simulink model "UKF_MPCwithDISTandRefer"  (R2016a)
settings: Solver=ode3  SolverMode=SingleTasking  StartTime=0.0  StopTime=32400  FixedStep=Ts  RelTol=1e-3
values from neighbouring files (symbols this model uses):
  R = log(D_ins_out / D_pipe) / (2 * pi * K * L/segments)    [Custom_pipe.m]    (also in ini_pipe_detailed.m = log(D_ins_out / D_pipe) / (2 * pi* K * L/segments))
undefined symbols (not defined in the file or in its folder): Nc, P_0, Q, Ts, x0_plant, x_s0, y_max, y_min
settings Model: Creator=saif  LastModifiedBy=lenovo
settings DataIOCC: LimitDataPoints=on  SaveFormat=Array
settings OptimizationCC: BlockReduction=off  BooleanDataType=off
settings DebuggingCC: SaveWithParameterizedLinksMsg=none  UnderspecifiedInitializationDetection=Classic  MergeDetectMultiDrivingBlocksExec=none  SignalResolutionControl=TryResolveAllWithWarning
settings HardwareCC: ProdBitPerPointer=32  ProdLargestAtomicFloat=None  ProdIntDivRoundTo=Undefined  ProdEndianess=Unspecified  ProdWordSize=32  ProdHWDeviceType=32-bit Generic  TargetUnknown=on
settings ModelReferenceCC: PropagateSignalLabelsOutOfModel=off
settings ConfigComp: CovModelRefEnable=Off  CovSFcnEnable=off

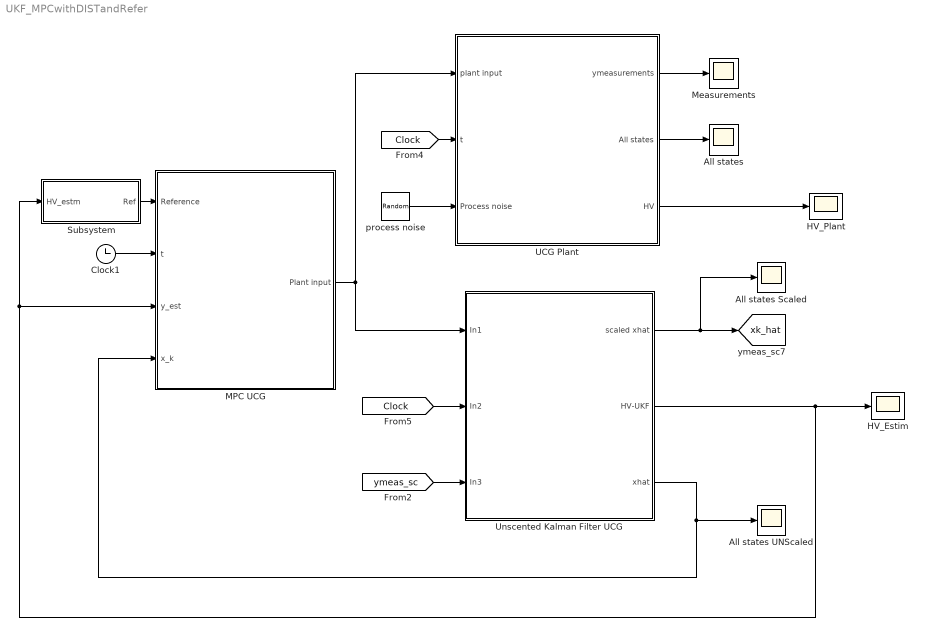
== system UKF_MPCwithDISTandRefer ==
  All states : Scope
  All states Scaled : Scope
  All states UNScaled : Scope
  Clock1 : Clock
  HV_Estim : Scope
  HV_Plant : Scope
  MPC UCG : Subsystem
  Measurements : Scope
  Subsystem : Subsystem
  UCG Plant : Subsystem
  Unscented Kalman Filter UCG : Subsystem
  process noise : RandomNumber  Variance=1e-4  SampleTime=Ts
  tag scope: xk_hat=global
  wires:
  process noise/1 -> UCG Plant/3(Process noise)
  UCG Plant/1(ymeasurements) -> Measurements/1
  UCG Plant/2(All states) -> All states/1
  Unscented Kalman Filter UCG/1(scaled xhat) -> All states Scaled/1, [xk_hat]
  Subsystem/1(Ref) -> MPC UCG/1(Reference)
  Clock1/1 -> MPC UCG/2(t)
  [Clock] -> UCG Plant/2(t)
  [Clock] -> Unscented Kalman Filter UCG/2(In2)
  UCG Plant/3(HV) -> HV_Plant/1
  Unscented Kalman Filter UCG/2(HV-UKF) -> Subsystem/1(HV_estm), MPC UCG/3(y_est), HV_Estim/1
  Unscented Kalman Filter UCG/3(xhat) -> All states UNScaled/1, MPC UCG/4(x_k)
  MPC UCG/1(Plant input) -> UCG Plant/1(plant input), Unscented Kalman Filter UCG/1(In1)
  [ymeas_sc] -> Unscented Kalman Filter UCG/3(In3)

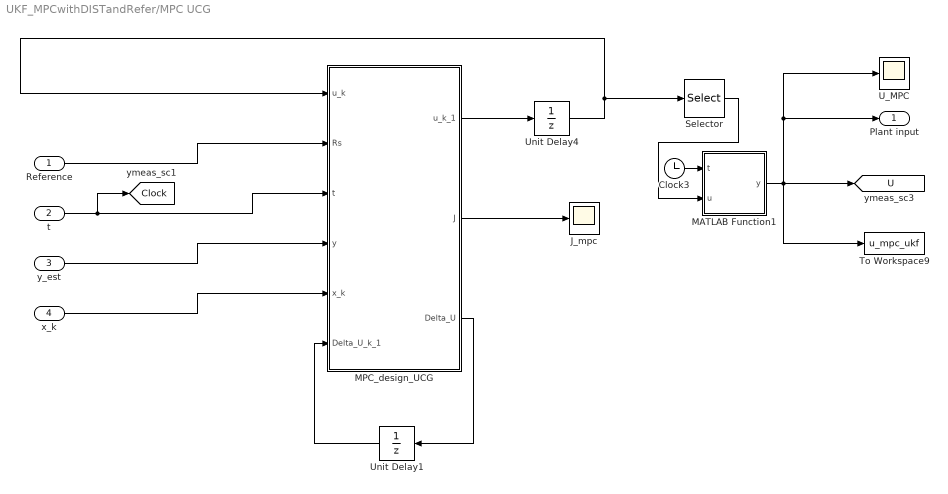
== system UKF_MPCwithDISTandRefer/MPC UCG ==
  Reference : Inport
  t : Inport  Port=2
  y_est : Inport  Port=3
  x_k : Inport  Port=4
  Clock3 : Clock
  J_mpc : Scope
  MATLAB Function1 : MATLAB Function  TreatAsAtomicUnit=on
  MPC_design_UCG : MATLAB Function  TreatAsAtomicUnit=on
  Selector : Selector  InputPortWidth=Nc  IndexOptions=Index vector (dialog)  Indices=[1]  OutputSizes=1
  To Workspace9 : ToWorkspace  VariableName=u_mpc_ukf  SampleTime=-1
  U_MPC : Scope
  Unit Delay1 : UnitDelay  InitialCondition=2e-4*ones(Nc,1)  SampleTime=-1
  Unit Delay4 : UnitDelay  InitialCondition=2e-4*ones(Nc,1)  SampleTime=-1
  Plant input : Outport
  tag scope: Clock=global, U=global
  wires:
  MATLAB Function1/1(y) -> To Workspace9/1, U_MPC/1, Plant input/1, [U]
  MPC_design_UCG/1(u_k_1) -> Unit Delay4/1
  Unit Delay4/1 -> MPC_design_UCG/1(u_k), Selector/1
  Selector/1 -> MATLAB Function1/2(u)
  Clock3/1 -> MATLAB Function1/1(t)
  t/1 -> [Clock], MPC_design_UCG/3(t)
  Reference/1 -> MPC_design_UCG/2(Rs)
  y_est/1 -> MPC_design_UCG/4(y)
  x_k/1 -> MPC_design_UCG/5(x_k)
  MPC_design_UCG/2(J) -> J_mpc/1
  MPC_design_UCG/3(Delta_U) -> Unit Delay1/1
  Unit Delay1/1 -> MPC_design_UCG/6(Delta_U_k_1)

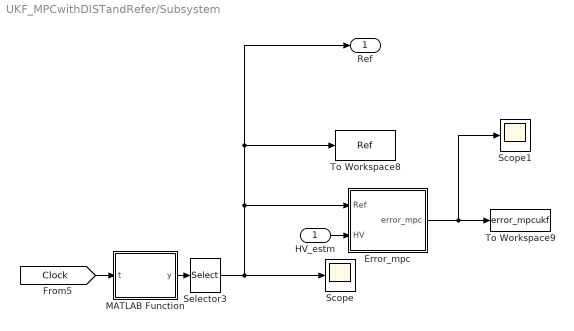
== system UKF_MPCwithDISTandRefer/Subsystem ==
  HV_estm : Inport
  Error_mpc : MATLAB Function  TreatAsAtomicUnit=on
  MATLAB Function : MATLAB Function  TreatAsAtomicUnit=on
  Scope : Scope
  Scope1 : Scope
  Selector3 : Selector  InputPortWidth=4  IndexOptions=Index vector (dialog)  Indices=[1]  OutputSizes=1
  To Workspace8 : ToWorkspace  VariableName=Ref  SampleTime=-1
  To Workspace9 : ToWorkspace  VariableName=error_mpcukf  SampleTime=-1
  Ref : Outport
  wires:
  HV_estm/1 -> Error_mpc/2(HV)
  Error_mpc/1(error_mpc) -> Scope1/1, To Workspace9/1
  [Clock] -> MATLAB Function/1(t)
  MATLAB Function/1(y) -> Selector3/1
  Selector3/1 -> Error_mpc/1(Ref), Ref/1, To Workspace8/1, Scope/1

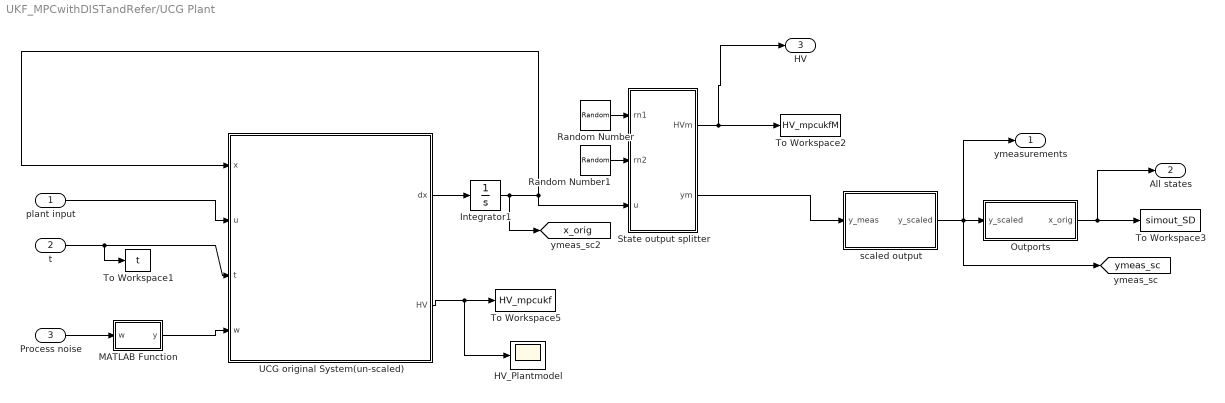
== system UKF_MPCwithDISTandRefer/UCG Plant ==
  plant input : Inport
  t : Inport  Port=2
  Process noise : Inport  Port=3
  HV_Plantmodel : Scope
  Integrator1 : Integrator  InitialCondition=x0_plant
  MATLAB Function : MATLAB Function  TreatAsAtomicUnit=on
  Outports : Subsystem
  Random Number : RandomNumber  Variance=4e-4
  Random Number1 : RandomNumber  Variance=4e-4
  State output splitter : MATLAB Function  TreatAsAtomicUnit=on
  To Workspace1 : ToWorkspace  VariableName=t  SampleTime=-1
  To Workspace2 : ToWorkspace  VariableName=HV_mpcukfM  SampleTime=-1
  To Workspace3 : ToWorkspace  VariableName=simout_SD  SampleTime=-1
  To Workspace5 : ToWorkspace  VariableName=HV_mpcukf  SampleTime=-1
  UCG original System(un-scaled) : MATLAB Function  TreatAsAtomicUnit=on
  scaled output : MATLAB Function  TreatAsAtomicUnit=on
  ymeasurements : Outport
  All states : Outport  Port=2
  HV : Outport  Port=3
  tag scope: x_orig=global, ymeas_sc=global
  wires:
  State output splitter/2(ym) -> scaled output/1(y_meas)
  scaled output/1(y_scaled) -> ymeasurements/1, Outports/1(y_scaled), [ymeas_sc]
  Outports/1(x_orig) -> All states/1, To Workspace3/1
  Integrator1/1 -> [x_orig], State output splitter/3(u), UCG original System(un-scaled)/1(x)
  Process noise/1 -> MATLAB Function/1(w)
  UCG original System(un-scaled)/1(dx) -> Integrator1/1
  MATLAB Function/1(y) -> UCG original System(un-scaled)/4(w)
  t/1 -> To Workspace1/1, UCG original System(un-scaled)/3(t)
  plant input/1 -> UCG original System(un-scaled)/2(u)
  UCG original System(un-scaled)/2(HV) -> HV_Plantmodel/1, To Workspace5/1
  Random Number/1 -> State output splitter/1(rn1)
  Random Number1/1 -> State output splitter/2(rn2)
  State output splitter/1(HVm) -> To Workspace2/1, HV/1

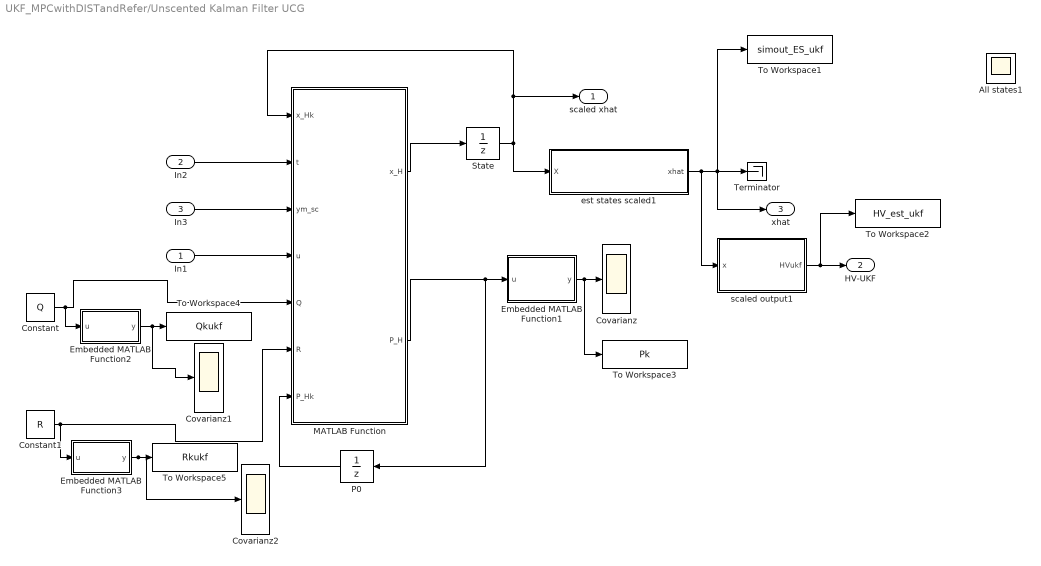
== system UKF_MPCwithDISTandRefer/Unscented Kalman Filter UCG ==
  In1 : Inport
  In2 : Inport  Port=2
  In3 : Inport  Port=3
  All states1 : Scope
  Constant : Constant  Value=Q
  Constant1 : Constant  Value=R
  Covarianz : Scope
  Covarianz1 : Scope
  Covarianz2 : Scope
  Embedded MATLAB Function1 : MATLAB Function  TreatAsAtomicUnit=on
  Embedded MATLAB Function2 : MATLAB Function  TreatAsAtomicUnit=on
  Embedded MATLAB Function3 : MATLAB Function  TreatAsAtomicUnit=on
  MATLAB Function : MATLAB Function  TreatAsAtomicUnit=on
  P0 : UnitDelay  InitialCondition=P_0  SampleTime=-1
  State : UnitDelay  InitialCondition=x_s0  SampleTime=-1
  Terminator : Terminator
  To Workspace1 : ToWorkspace  VariableName=simout_ES_ukf  SampleTime=-1
  To Workspace2 : ToWorkspace  VariableName=HV_est_ukf  SampleTime=-1
  To Workspace3 : ToWorkspace  VariableName=Pk  SampleTime=-1
  To Workspace4 : ToWorkspace  VariableName=Qkukf  SampleTime=-1
  To Workspace5 : ToWorkspace  VariableName=Rkukf  SampleTime=-1
  est states scaled1 : MATLAB Function  TreatAsAtomicUnit=on
  scaled output1 : MATLAB Function  TreatAsAtomicUnit=on
  scaled xhat : Outport
  HV-UKF : Outport  Port=2
  xhat : Outport  Port=3
  wires:
  Embedded MATLAB Function1/1(y) -> To Workspace3/1, Covarianz/1
  State/1 -> est states scaled1/1(X), scaled xhat/1, MATLAB Function/1(x_Hk)
  In3/1 -> MATLAB Function/3(ym_sc)
  P0/1 -> MATLAB Function/7(P_Hk)
  MATLAB Function/2(P_H) -> P0/1, Embedded MATLAB Function1/1(u)
  MATLAB Function/1(x_H) -> State/1
  Constant1/1 -> Embedded MATLAB Function3/1(u), MATLAB Function/6(R)
  In2/1 -> MATLAB Function/2(t)
  est states scaled1/1(xhat) -> scaled output1/1(x), xhat/1, To Workspace1/1, Terminator/1
  In1/1 -> MATLAB Function/4(u)
  scaled output1/1(HVukf) -> To Workspace2/1, HV-UKF/1
  Constant/1 -> Embedded MATLAB Function2/1(u), MATLAB Function/5(Q)
  Embedded MATLAB Function3/1(y) -> Covarianz2/1, To Workspace5/1
  Embedded MATLAB Function2/1(y) -> Covarianz1/1, To Workspace4/1

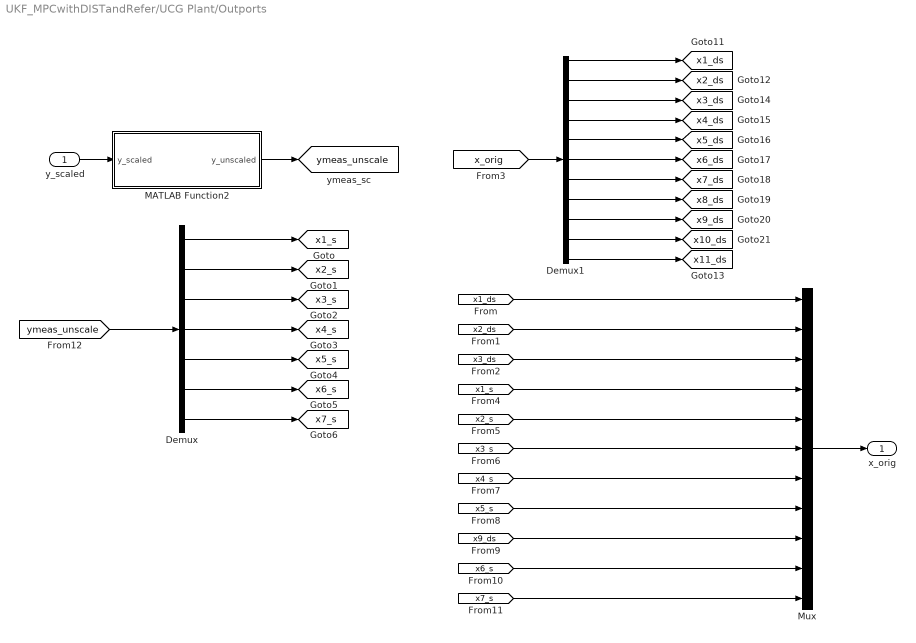
== system UKF_MPCwithDISTandRefer/UCG Plant/Outports ==
  y_scaled : Inport
  Demux : Demux  Outputs=7
  Demux1 : Demux  Outputs=11
  MATLAB Function2 : MATLAB Function  TreatAsAtomicUnit=on
  Mux : Mux  Inputs=11
  x_orig : Outport
  tag scope: x10_ds=global, x11_ds=global, x1_ds=global, x1_s=global, x2_ds=global, x2_s=global, x3_ds=global, x3_s=global, x4_ds=global, x4_s=global, x5_ds=global, x5_s=global, x6_ds=global, x6_s=global, x7_ds=global, x7_s=global, x8_ds=global, x9_ds=global, ymeas_unscale=global
  wires:
  [x1_ds] -> Mux/1
  [x2_ds] -> Mux/2
  [x3_ds] -> Mux/3
  [x1_s] -> Mux/4
  [x2_s] -> Mux/5
  [x3_s] -> Mux/6
  [x4_s] -> Mux/7
  [x5_s] -> Mux/8
  [x9_ds] -> Mux/9
  [x6_s] -> Mux/10
  [x7_s] -> Mux/11
  Mux/1 -> x_orig/1
  y_scaled/1 -> MATLAB Function2/1(y_scaled)
  MATLAB Function2/1(y_unscaled) -> [ymeas_unscale]
  Demux/5 -> [x5_s]
  Demux/7 -> [x7_s]
  Demux/6 -> [x6_s]
  Demux/4 -> [x4_s]
  Demux/1 -> [x1_s]
  Demux/2 -> [x2_s]
  Demux/3 -> [x3_s]
  [ymeas_unscale] -> Demux/1
  Demux1/3 -> [x3_ds]
  Demux1/2 -> [x2_ds]
  Demux1/1 -> [x1_ds]
  Demux1/4 -> [x4_ds]
  [x_orig] -> Demux1/1
  Demux1/11 -> [x11_ds]
  Demux1/9 -> [x9_ds]
  Demux1/10 -> [x10_ds]
  Demux1/8 -> [x8_ds]
  Demux1/6 -> [x6_ds]
  Demux1/7 -> [x7_ds]
  Demux1/5 -> [x5_ds]

== matlab function UKF_MPCwithDISTandRefer/Unscented Kalman Filter UCG/Embedded MATLAB Function1 ==
  data: u input; y output
function y = fcn(u)
% This block supports the Embedded MATLAB subset.
% See the help menu for details. 

y = sqrt(diag(u));

== matlab function UKF_MPCwithDISTandRefer/Unscented Kalman Filter UCG/MATLAB Function ==
  data: x_Hk input; t input; ym_sc input; u input; x_H output; Q input; R input; P_Hk input; P_H output
function [x_H,P_H] = fcn(x_Hk, t, ym_sc, u, Q, R, P_Hk)
%#codegen
Ts = 2.5;
%% Eingänge
%% Unscented Kalman Filter
% Anweisungen:
% - an das jeweilige Modell müssen zwei Punkte angepasst werden:
%   (II) die diskrete Systemdarstellung für die Sigmapunkte der Zustände
%   (V) die Ausgangsgleichungen für die Sigmapunkte der Messungen
% (Kennzeichnung der Stellen durch %%%%%%%%%%%% )
% - optional können die Skalierungsfaktoren al, ka und be angepasst werden
% - alle restlichen Punkte sollten unverändert bleiben
% - Notation: H = Hut, M = minus, k = aktueller Zeitschritt, km1 = vorheriger
% Zeitschritt, sigX/sigY = Matrizen der Sigmapunkte um X/Y
nx = size(x_Hk,1); %Anzahl Zustände
ny = size(ym_sc,1); %Anzahl Messwerte
nsig = 2*nx+1; %Anzahl Sigmas
%Time update
%% Skalierungsfaktoren und Gewichtungen
% 0<=alpha<=1,kontrolliert Größe der Sigmapunkt-Verteilung, standard: 1e-3
alpha   = 1;%5e-1;
%kappa>= 0 garantiert positiv semidefinite Kovarianzmatrix, standard: 0
kappa   = 0;
%beta >= 0, "incorporate knowledge of the higher order moments of the distribution", standard: 2
beta    = 2;
%scaling factor
lambda=alpha^2*(nx+kappa)-nx;
%scaling factor
c=nx+lambda;
%weights for means
Wm=[lambda/c 1/(2*c)+zeros(1,2*nx)];
Wc=Wm;
%weights for covariance
Wc(1)=Wc(1)+(1-alpha^2+beta);
%% Time update
%% (I) Sigma Punkte für aktuelle Zustände
sigX_km1 = sigmas2(x_Hk,P_Hk,c);
%% (II) Nichtlineare Systemdarstellung xp = f(x,u)
sigX_kkm1 = zeros(nx,nsig);
for k = 1:nsig
    %%%%%%%%%%%% diskrete System representation in explicit Euler form:
    %%x_(k+1) = x_(k) + Ts*f(x_(k),u_(k),z)
    %%%%%%%%%%%% Heun's form:
    %%x_(k+1) = x_(k) + Ts [(1/2*f(x_(k),u_(k),z))+1/2*f(x_(k)+Ts*f(x_(k),u_(k),z),u_(k),z)]
    %% Heun Verfahren:
    f = dgl(sigX_km1(:,k), u, t);   % f(x_k,u_k)
    % update x_k + Ts*f(x_k,u_k)
    X_k = sigX_km1(:,k);
    Xk_1 = X_k + Ts*f;
    f_1 = dgl(Xk_1, u, t);    % f(x_k + Ts*f(x_k,u_k),u_k)
    XK_1 = X_k + Ts * (1/2*f + 1/2*f_1);
    sigX_kkm1(:,k) = XK_1;
end
%% (III) State prediction
xHM_k = zeros(nx,1);
for k=1:nsig
    xHM_k = xHM_k+Wm(k).*sigX_kkm1(:,k);
end
%% (IV) Covariance matrix - Prediction
PM_xk = (sigX_kkm1-xHM_k(:,ones(1,nsig)))*diag(Wc)*(sigX_kkm1-xHM_k(:,ones(1,nsig))).' + Q;
%% Measurement update
%% (V) Sigmapunkte der Messungen (Transformation y_m=h(x))
sigY_kkm1 = zeros(ny,nsig);
for k = 1:nsig
    %%%%%%%%%%%% output equations
    % [rho_coal rho_char T_s C_CO C_CO2 C_H2 C_CH4 C_Tar C_H2O C_O2 C_N2]
    sigY_kkm1(1,k) = sigX_kkm1(4,k);
    sigY_kkm1(2,k) = sigX_kkm1(5,k);
    sigY_kkm1(3,k) = sigX_kkm1(6,k);
    sigY_kkm1(4,k) = sigX_kkm1(7,k);
    sigY_kkm1(5,k) = sigX_kkm1(8,k);
    sigY_kkm1(6,k) = sigX_kkm1(10,k);
    sigY_kkm1(7,k) = sigX_kkm1(11,k);
end
%% (VI) Measurement prediction
yHM_k = zeros(ny,1);
for k=1:nsig
    yHM_k = yHM_k+Wm(k).*sigY_kkm1(:,k);
end
%% (VII) Covariance matrix of estimated measurements
P_yk = (sigY_kkm1-yHM_k(:,ones(1,nsig)))*diag(Wc)*(sigY_kkm1-yHM_k(:,ones(1,nsig))).' + R;
%% (VIII) Cross-covarariance between estimated states and measurements
P_xkyk = (sigX_kkm1-xHM_k(:,ones(1,nsig)))*diag(Wc)*(sigY_kkm1-yHM_k(:,ones(1,nsig))).';
%% (IX) Update of states and covariance matrix
% mit bekannten Kalman Filter Gleichungen
L_k  = P_xkyk/P_yk; %Verstärkungsmatrix
xH_k = xHM_k+L_k*(ym_sc-yHM_k);
P_xk = PM_xk - L_k*P_yk*L_k.';
x_H = xH_k;
P_H = P_xk;
HV=zeros(1,1);
end

function f = dgl(sigX_km, u, t)
rho_coal_sc     = sigX_km(1);
rho_char_sc     = sigX_km(2);
Ts_sc           = sigX_km(3);
C_CO_sc         = sigX_km(4);
C_CO2_sc        = sigX_km(5);
C_H2_sc         = sigX_km(6);
C_CH4_sc        = sigX_km(7);
C_Tar_sc        = sigX_km(8);
C_H2O_sc        = sigX_km(9);
C_O2_sc         = sigX_km(10);
C_N2_sc         = sigX_km(11);
x_sc = [rho_coal_sc;    rho_char_sc;    Ts_sc;...
    C_CO_sc;        C_CO2_sc;       C_H2_sc;...
    C_CH4_sc;       C_Tar_sc;       C_H2O_sc;...
    C_O2_sc;        C_N2_sc];
%% unscaled states
% rho_coal = x(1);
% rho_char = x(2);
% T_s      = x(3);
% C_CO     = x(4);
% C_CO2    = x(5);
% C_H2     = x(6);
% C_CH4    = x(7);
% C_Tar    = x(8);
% C_H2O    = x(9);
% C_O2     = x(10);
% C_N2     = x(11);
%% Parameters of Plant
st_oxy  = 5;
oxygen  = 0.154;
steam   = 0.154*st_oxy;
nitrogen = 1-oxygen-steam;
Ha      = 282.8;          % KJ*mol-1, heat of combustion of CO
Hb      = 283.6;          % KJ*mol-1, heat of combustion of H2
Hc      = 836.16;         % KJ*mol-1, heat of combustion of CH4
L       = 100;            % cm, Reactor length
ug      = 1;              % cm*s-1, gas burst velocity
ht      = 0.001;          % cal*s-1*cm-3*k-1, heat transfer coefficient
ky      = 0.1*ht;
H2      = -93929 ;        % cal*mol-1, heat of char oxidation reaction
H3      = 31309.7;        % cal*mol-1, heat of steam gasification reaction
cs      = 7.3920;         % cal*cm-3*k-1, total solid phase heat capacity
MW_Coal = 13.106;         % g*mol-1, molecular weight of coal
MW_Char = 12.47;          % g*mol-1, molecular weight of char
P       = 4.83;           % atm, pressure
beta    = 7e-6;

%%
A       = 1/cs;
%% Control input
U     = u;
%% converting scaled states to unsclaed
rhoCoal_max = 0.4996;
rhoChar_max= 0.2161;
Ts_max= 873.368;
CO_max=0.0127;
CO2_max=0.0131;
H2_max=0.0150;
CH4_max=0.0015;
Tar_max=4.77e-4;
H2O_max=0.0561;
O2_max=0.0018;
N2_max=0.0075;

x_max = [rhoCoal_max;rhoChar_max;Ts_max;CO_max;CO2_max;H2_max;CH4_max;Tar_max;H2O_max;O2_max;N2_max];
x_min = [0.00001;0.00002;450;0;0;0;0;0;0;0;0];

for i=1:11
    if (x_sc(i)< -((x_min(i))/(x_max(i)-x_min(i))))
        x_sc(i) = -(x_min(i))/(x_max(i)-x_min(i));
    end
end
%     x(x<0)=0;
x_der = zeros(11,1);
for i=1:1:11
    x_der(i) = 1./(x_max(i)-x_min(i));
end
x = zeros(11,1); % unscaled states
for i=1:1:11
    x(i) = x_sc(i)*(x_max(i)-x_min(i))+x_min(i);
end
% x(x<0)=0;
%% molar fraction
CT = x(4)+x(5)+x(6)+x(7)+x(8)+x(10)+x(11);
mf_CO   = x(4)./CT;
mf_CO2  = x(5)./(CT);
mf_H2   = x(6)./CT;
mf_CH4  = x(7)./CT;
mf_Tar  = x(9)./(CT);
mf_H2O  = x(9)./(CT+x(9));
mf_O2   = x(10)./(CT);
mf_N2   = x(11)./(CT);
mf_O2_2 = x(10)./(CT+x(9));
HV      = Ha*mf_CO+Hb*mf_H2+Hc*mf_CH4;
l       = [0   100 500 1000 5000 10000 20000 30000 50000];
k       = [450 550 800 1100 1000 900   850   850   850];
T       = interp1(l,k,t,'pchip');
R1      = (0.3*x(1)*exp(-6039/x(3)))/MW_Coal;
Rc2     = (9.55e7*x(2)*P*mf_O2_2*exp(-22142/x(3)))/ (MW_Char*x(3)^0.5);
Rm2     = ky*mf_O2_2;
R2      = 120*(1/((1/Rc2)+(1/Rm2)));
Rc3     = (2*x(2)*mf_H2O^2*P^2*exp(5.052-12908/x(3)))/(MW_Char*(1e-5*mf_H2O*P+exp(-22.216 + 24880/x(3)))^2);
Rm3     = ky*mf_H2O;
R3      = 3*10^4*(1/((1/Rc3)+(1/Rm3)));
%% time-derivative of scaled states
% g*cm-3*s-1, coal density
x1dot  = x_der(1)*(-MW_Coal*R1);
% g*cm-3*s-1, char density
x2dot  = x_der(2)*(MW_Char*(0.766*R1-R2-R3));
% k*s-1, solid temperature
x3dot  = x_der(3)*(A*(ht*(T-x(3))-H2*R2-H3*R3));
% CO
x4dot  = x_der(4)*(0.008*R1+R3-x(4)*beta);
% CO2
x5dot  = x_der(5)*(0.058*R1+R2-x(5)*beta);
% H2
x6dot  = x_der(6)*(0.083*R1+R3-x(6)*beta);
% CH4
x7dot  = x_der(7)*(0.044*R1-x(7)*beta);
% Tar
x8dot  = x_der(8)*((0.124/9)*R1-x(8)*beta);
% H2O
x9dot  = x_der(9)*(0.055*R1+0.075*R2-0.925*R3+U*steam/L-x(9)*beta);
% O2
x10dot = x_der(10)*(-1.02*R2+U*oxygen/L-x(10)*beta);
% N2
x11dot = x_der(11)*(U*nitrogen/L-x(11)*beta);
f = [x1dot;x2dot;x3dot;x4dot;x5dot;x6dot;x7dot;x8dot;x9dot;x10dot;x11dot];
end

== matlab function UKF_MPCwithDISTandRefer/UCG Plant/UCG original System(un-scaled) ==
  data: x input; u input; t input; dx output; HV output; w input
function [dx,HV] = fcn(x,u,t,w)
%#codegen

% dp_dt = r*p*(1-p/k);
dx = zeros(11,1);
dxx=zeros(11,1);
st_oxy  = 5;
oxygen  = 0.154;
steam   = 0.154*st_oxy;
nitrogen = 1-oxygen-steam;
Ha      = 282.8;          %KJ*mol-1, heat of combustion of CO
Hb      = 283.6;          %KJ*mol-1, heat of combustion of H2
Hc      = 836.16;         %KJ*mol-1, heat of combustion of CH4
L       = 100;            %cm, Reactor length
ug      = 1;              %cm*s-1, gas burst velocity
ht      = 0.001;                  %cal*s-1*cm-3*k-1, heat transfer coefficient
ky      = 0.1*ht;
H2      = -93929 ;               % cal*mol-1, heat of char oxidation reaction
H3      = 31309.7;               % cal*mol-1, heat of steam gasification reaction
cs      = 7.3920;                  % cal*cm-3*k-1, total solid phase heat capacity
MW_Coal = 13.106;            % g*mol-1, molecular weight of coal
MW_Char = 12.47;            % g*mol-1, molecular weight of char
% P       =4.83;                      %atm, pressure
P       =4.83;                      %atm, pressure
A       = 1/cs;
beta    = 7e-6;
HV      = 0;
%% Parametric variation
P    = P+0.02*P;
beta = beta-0.02*beta;
ht   = ht+0.02*ht;
cs   = cs-0.02*cs;
%% States evaluaion
x(x<0)=0;
CT = x(4)+x(5)+x(6)+x(7)+x(8)+x(10)+x(11);

mf_CO   = x(4)./(CT);
%mf_CO2  = x(5)./(CT);
mf_H2   = x(6)./(CT);
mf_CH4  = x(7)./(CT);
%mf_Tar  = x(9)./(CT);
mf_H2O  = x(9)./(CT+x(9));
%mf_O2   = x(10)./(CT);
%mf_N2   = x(11)./(CT);
mf_O2_2 = x(10)./(CT+x(9));

HV      = Ha*mf_CO+Hb*mf_H2+Hc*mf_CH4;

l       =[0   100 500 1000 5000 10000 20000 30000 50000];
k       =[450 550 800 1100 1000 900   850   850   850];
T       = interp1(l,k,t,'pchip');   

dd = [0     20000     26300     32400   50000];
dy = [0     0         3e-5    0    0];

delta = interp1(dd,dy,t,'pchip');
R1      = (0.3*x(1)*exp(-6039/x(3)))/MW_Coal;
Rc2     = (9.55e7*x(2)*P*mf_O2_2*exp(-22142/x(3)))/ (MW_Char*x(3)^0.5);
Rm2     = ky*mf_O2_2;
R2      = 120*(1/((1/Rc2)+(1/Rm2)));
Rc3     = (2*x(2)*mf_H2O^2*P^2*exp(5.052-12908/x(3)))/(MW_Char*(1e-5*mf_H2O*P+exp(-22.216 + 24880/x(3)))^2);
Rm3     = ky*mf_H2O;
R3      = 3*10^4*(1/((1/Rc3)+(1/Rm3)));

U      = u;
x1dot  = -MW_Coal*R1;                                                 %g*cm-3*s-1, derivative of coal density
x2dot  =  MW_Char*(0.766*R1-R2-R3);                                   %g*cm-3*s-1, derivative of char density
x3dot  =  A*(ht*(T-x(3))-H2*R2-H3*R3);                                %k*s-1, derivative of solid temperature
x4dot  =  0.008*R1+R3-x(4)*beta;                                      %CO
x5dot  =  0.058*R1+R2-x(5)*beta;                                      %CO2
x6dot  =  0.083*R1+R3-x(6)*beta;                                      %H2
x7dot  =  0.044*R1-x(7)*beta;                                         %methane
x8dot  =  (0.124/9)*R1-x(8)*beta;                                     %Tar
x9dot  =  0.055*R1+0.075*R2-0.925*R3+U*steam/L-x(9)*beta+delta/L;             %steam
x10dot = -1.02*R2+U*oxygen/L-x(10)*beta;                              %O2
x11dot =  U*nitrogen/L-x(11)*beta;                                    %N2
dxx = [x1dot;x2dot;x3dot;x4dot;x5dot;x6dot;x7dot;x8dot;x9dot;x10dot;x11dot];

dx=dxx+dxx.*w;
% dx = [dx1;dx2];

== matlab function UKF_MPCwithDISTandRefer/Unscented Kalman Filter UCG/est states scaled1 ==
  data: X input; xhat output
function xhat = EstStates_UnScaled(X)
%%
rho_coal_sc = X(1);
rho_char_sc = X(2);
Ts_sc       = X(3);
C_CO_sc     = X(4);
C_CO2_sc    = X(5);
C_H2_sc     = X(6);
C_CH4_sc    = X(7);
C_Tar_sc    = X(8);
C_H2O_sc    = X(9);
C_O2_sc     = X(10);
C_N2_sc     = X(11);
%% max value
rho_coalmax = 0.4996;
rho_charmax = 0.2161;
Ts_max      = 873.368;
C_COmax     = 0.0127;
C_CO2max    = 0.0131;
C_H2max     = 0.0150;
C_CH4max    = 0.0015;
C_Tarmax    = 4.77e-4;
C_H2Omax    = 0.0561;
C_O2max     = 0.0018;
C_N2max     = 0.0075;
%% min value
rho_coalmin = 0.00001;
rho_charmin = 0.00002;
Ts_min      = 450;
C_COmin     = 0;
C_CO2min    = 0;
C_H2min     = 0;
C_CH4min    = 0;
C_Tarmin    = 0;
C_H2Omin    = 0;
C_O2min     = 0;
C_N2min     = 0;
%% states unscaled
rho_coal    = (rho_coalmax  -  rho_coalmin  ) * rho_coal_sc + rho_coalmin;
rho_char    = (rho_charmax  -  rho_charmin  ) * rho_char_sc + rho_charmin;
Ts          = (Ts_max  -   Ts_min   ) * Ts_sc     + Ts_min;
C_CO        = (C_COmax  -  C_COmin  ) * C_CO_sc   + C_COmin;
C_CO2       = (C_CO2max -  C_CO2min ) * C_CO2_sc  + C_CO2min;
C_H2        = (C_H2max  -  C_H2min  ) * C_H2_sc   + C_H2min;
C_CH4       = (C_CH4max -  C_CH4min ) * C_CH4_sc  + C_CH4min;
C_Tar       = (C_Tarmax -  C_Tarmin ) * C_Tar_sc  + C_Tarmin;
C_H2O       = (C_H2Omax  - C_H2Omin ) * C_H2O_sc  + C_H2Omin;
C_O2        = (C_O2max  -  C_O2min  ) * C_O2_sc   + C_O2min;
C_N2        = (C_N2max  -  C_N2min  ) * C_N2_sc   + C_N2min;
%%
xhat = [rho_coal;rho_char;Ts;C_CO;C_CO2;C_H2;C_CH4;C_Tar;C_H2O;C_O2;C_N2];
end

== matlab function UKF_MPCwithDISTandRefer/UCG Plant/Outports/MATLAB Function2 ==
  data: y_scaled input; y_unscaled output; y_max parameter; y_min parameter
function y_unscaled   = fcn(y_scaled,y_max,y_min)
%#codegen

y_unscaled=zeros(7,1);

for i=1:length(y_unscaled )
y_unscaled (i) = y_scaled(i)*(y_max(i)-y_min(i))+y_min(i);
end

== matlab function UKF_MPCwithDISTandRefer/MPC UCG/MPC_design_UCG ==
  data: u_k input; Rs input; t input; y input; x_k input; Ts parameter; Delta_U_k_1 input; u_k_1 output; J output; Delta_U output
% function [u_k_1, x_kn,Aa,B,C,R_s,R_hat,Delta_U] = fcn(u_k,Rs,t,y,x_k,Ts)
function [u_k_1,J,Delta_U]  = fcn(u_k,Rs,t,y,x_k,Ts,Delta_U_k_1)
%  global x_kn R_hat R_s B Aa C Np Nc
% coder.extrinsic('quadprog');
J = 0;
coder.extrinsic('fmincon');
coder.extrinsic('MPC_UCG');
coder.extrinsic('optimoptions');
coder.extrinsic('tic');
coder.extrinsic('toc');
% tic
%%%%%%% MPC design Parameters
%% Cheange Np and Nc here as well
Nc=5;
Np=5;

rw=1;%%% 
% Rs= 2.032454207540577e+02;%t=20000sec %203.2400%t=20010; %%%% Reference 
% Rs=200;
R_s=Rs*ones(Np,1); % For reference signal
R_hat=rw*eye(Nc,Nc); % For bounded control input
x_kn=zeros(12,1);
Aa=zeros(12,12);
B=zeros(12,1);
C=zeros(1,12);
% Delta_U=zeros(Nc,1);
Delta_U=Delta_U_k_1;
if t<=20000
    u_k_1=[1*2e-4;1*2e-4*ones(Nc-1,1)];

else
%% Discretized Plant
x=x_k;
%#codegen
% dx = zeros(4,1);
A_op = zeros(11,11);
B_sys = zeros(11,2);
C_sys=zeros(1,11);

f_x   = zeros(11,1);
dx_k_1=zeros(11,1);
% x_kn=zeros(12,1);
X=zeros(Nc,1);
% J=0;
% Delta_U=zeros(Nc,1);
Delta_U=Delta_U_k_1;
%% parameters
ht      = 0.001;                  %cal*s-1*cm-3*k-1, heat transfer coefficient
ky      = 0.1*ht;
H2      = -93929 ;               % cal*mol-1, heat of char oxidation reaction
H3      = 31309.7;               % cal*mol-1, heat of steam gasification reaction
cs      = 7.3920;                  % cal*cm-3*k-1, total solid phase heat capacity
MW_Coal = 13.106;            % g*mol-1, molecular weight of coal
MW_Char = 12.47;            % g*mol-1, molecular weight of char
P       =4.83;                      %atm, pressure
A       = 1/cs;
beta    = 7e-6;
Ha = 282.8;
Hb = 283.6;
Hc = 836.16;
 
%%
 
rho_coal = x(1);
rho_char = x(2);
T_s      = x(3);
C_CO     = x(4);
C_CO2    = x(5);
C_H2     = x(6);
C_CH4    = x(7);
C_Tar    = x(8);
C_H2O    = x(9);
C_O2     = x(10);
C_N2     = x(11);
 
 
%x_norm_f_2 = (rho_coal^2+rho_char^2+T_s^2+C_CO^2+C_CO2^2+C_H2^2+C_CH4^2+C_Tar^2+C_H2O^2+C_O2^2+C_N2^2);
 
 
x_norm_f_1 = (rho_coal^2+T_s^2);
x_norm_f_2 = (rho_coal^2+rho_char^2+T_s^2+C_CO2^2+C_CO^2+C_H2^2+C_CH4^2+C_Tar^2+C_H2O^2+C_O2^2+C_N2^2);
x_norm_f_3 = (rho_char^2+T_s^2+C_CO^2+C_CO2^2+C_H2^2+C_CH4^2+C_Tar^2+C_H2O^2+C_O2^2+C_N2^2);
x_norm_f_4 = (rho_coal^2+rho_char^2+T_s^2+C_CO^2+C_CO2^2+C_H2^2+C_CH4^2+C_Tar^2+C_H2O^2+C_O2^2+C_N2^2);
x_norm_f_5 = (rho_coal^2+rho_char^2+T_s^2+C_CO^2+C_CO2^2+C_H2^2+C_CH4^2+C_Tar^2+C_H2O^2+C_O2^2+C_N2^2);
x_norm_f_6 = (rho_coal^2+rho_char^2+T_s^2+C_CO^2+C_CO2^2+C_H2^2+C_CH4^2+C_Tar^2+C_H2O^2+C_O2^2+C_N2^2);
x_norm_f_7 = (rho_coal^2+T_s^2+C_CH4^2);
x_norm_f_8 = (rho_coal^2+T_s^2+C_Tar^2);
x_norm_f_9 = x_norm_f_4;
x_norm_f_10 = x_norm_f_3;
x_norm_f_11 = C_N2^2;
 
  
%%
l       =[0   100 500 1000 5000 10000 20000 30000 50000];
k       =[450 550 800 1100 1000 900   850   850   850];
T       = interp1(l,k,t,'pchip');    
 
N = Ha*C_CO+Hb*C_H2+Hc*C_CH4;
CT = x(4)+x(5)+x(6)+x(7)+x(8)+x(10)+x(11);
 
HV = N/CT;
 
 
mf_H2O  = x(9)./(CT+x(9));
mf_O2_2 = x(10)./(CT+x(9));
 
      
R1      = (0.3*x(1)*exp(-6039/x(3)))/MW_Coal;
Rc2     = (9.55e7*x(2)*P*mf_O2_2*exp(-22142/x(3)))/ (MW_Char*x(3)^0.5);
Rm2     = ky*mf_O2_2;
R2      = 120*(1/((1/Rc2)+(1/Rm2)));
Rc3     = (2*x(2)*mf_H2O^2*P^2*exp(5.052-12908/x(3)))/(MW_Char*(1e-5*mf_H2O*P+exp(-22.216 + 24880/x(3)))^2);
Rm3     = ky*mf_H2O;
R3      = 3*10^4*(1/((1/Rc3)+(1/Rm3)));
 
f_x(1,1)  = -MW_Coal*R1;                                %g*cm-3*s-1, derivative of coal density
f_x(2,1)  =  MW_Char*(0.766*R1-R2-R3);                  %g*cm-3*s-1, derivative of char density
f_x(3,1)  =  A*(ht*(-x(3))-H2*R2-H3*R3);              %k*s-1, derivative of solid temperature
f_x(4,1)  =  0.008*R1+R3-x(4)*beta;                                      %CO
f_x(5,1)  =  0.058*R1+R2-x(5)*beta;                                    %CO2
f_x(6,1)  =  0.083*R1+R3-x(6)*beta;                                 %H2
f_x(7,1)  =  0.044*R1-x(7)*beta;                                       %methane
f_x(8,1)  =  (0.124/9)*R1-x(8)*beta;                               %Tar
f_x(9,1)  =  0.055*R1+0.075*R2-0.925*R3-x(9)*beta;              %steam
f_x(10,1) = -1.02*R2-x(10)*beta;
f_x(11,1) =  -x(11)*beta;
 
 
 
%%
t1 = 1 / T_s;
t3 = exp(-(6039 * t1));
t6 = rho_coal * t3;
t9 = t1 * rho_coal * t3;
t12 = 0.1e1 / x_norm_f_1 * (0.3000000000e0 * t6 + 0.1811700000e4 * t9 + f_x(1,1));
t15 = T_s ^ 2;
t16 = 0.1e1 / t15;
t18 = rho_coal * t16 * t3;
t25 = 0.1e1 / rho_char;
t26 = 0.1e1 / C_O2;
t27 = t25 * t26;
t28 = C_CO + C_CO2 + C_H2 + C_CH4 + C_Tar + C_O2 + C_N2 + C_H2O;
t30 = exp(-(22142 * t1));
t31 = 0.1e1 / t30;
t32 = t28 * t31;
t33 = T_s ^ 0.5e0;
t34 = t32 * t33;
t40 = (0.2703435119e-7 * t27 * t34 + 0.1e5 * t26 * t28) ^ 2;
t41 = 0.1e1 / t40;
t42 = rho_char ^ 2;
t43 = 0.1e1 / t42;
t46 = t41 * t43 * t26 * t34;
t47 = 0.4045420312e-4 * t46;
t48 = C_H2O ^ 2;
t49 = 0.1e1 / t48;
t50 = t25 * t49;
t51 = t28 ^ 2;
t54 = exp(0.5052e1 - (12908 * t1));
t55 = 0.1e1 / t54;
t57 = 0.1e1 / t28;
t62 = exp(-0.22216e2 + (24880 * t1));
t63 = 0.483e-4 * C_H2O * t57 + t62;
t64 = t63 ^ 2;
t65 = t51 * t55 * t64;
t68 = 0.1e1 / C_H2O;
t72 = (0.2672650660e0 * t50 * t65 + 0.1e5 * t68 * t28) ^ 2;
t73 = 0.1e1 / t72;
t76 = t73 * t43 * t49 * t65;
t77 = 0.9998386119e5 * t76;
t80 = 0.1320417720e4 * t18;
t81 = T_s ^ (-0.15e1);
t85 = T_s ^ (-0.5e0);
t89 = -0.5985946040e-3 * t27 * t32 * t81 + 0.1351717560e-7 * t27 * t32 * t85;
t90 = t41 * t89;
t91 = 0.149640e4 * t90;
t92 = t50 * t51;
t97 = t55 * t63;
t103 = t73 * (-0.3449857472e4 * t92 * t55 * t64 * t16 - 0.1329910968e5 * t92 * t97 * t16 * t62);
t104 = 0.37410000e6 * t103;
t109 = 0.2703435119e-7 * t27 * t31 * t33;
t110 = 0.1e5 * t26;
t111 = t109 + t110;
t112 = t41 * t111;
t113 = 0.149640e4 * t112;
t117 = 0.5345301320e0 * t50 * t28 * t55 * t64;
t121 = 0.1e5 * t68;
t122 = t117 - 0.2581780538e-4 * t25 * t68 * t97 + t121;
t123 = t73 * t122;
t124 = 0.37410000e6 * t123;
t125 = t113 + t124;
t146 = -0.5345301320e0 * t25 / t48 / C_H2O * t65 + t117 + 0.5345301320e0 * t92 * t97 * (0.483e-4 * t57 - 0.483e-4 * C_H2O / t51) - 0.1e5 * t49 * t28 + t121;
t147 = t73 * t146;
t148 = 0.37410000e6 * t147;
t151 = C_O2 ^ 2;
t152 = 0.1e1 / t151;
t158 = -0.2703435119e-7 * t25 * t152 * t34 + t109 - 0.1e5 * t152 * t28 + t110;
t159 = t41 * t158;
t160 = 0.149640e4 * t159;
t164 = -0.2186484053e0 * t6 - rho_char * (-t47 - t77) - T_s * (t80 + t91 + t104) - C_CO * t125 - C_CO2 * t125 - C_H2 * t125 - C_CH4 * t125 - C_Tar * t125 - C_H2O * (t113 + t148) - C_O2 * (t160 + t124) - C_N2 * t125 + f_x(2,1);
t165 = 0.1e1 / x_norm_f_2 * t164;
t188 = 0.4122255801e-1 * t46;
t189 = 0.3396099448e8 * t76;
t193 = 0.1524821429e7 * t90;
t194 = 0.1270685877e9 * t103;
t197 = 0.1524821429e7 * t112;
t198 = 0.1270685877e9 * t123;
t199 = -t197 + t198;
t205 = 0.1270685877e9 * t147;
t208 = 0.1524821429e7 * t159;
t212 = -rho_char * (t188 - t189) - T_s * (-0.1352813853e-3 - t193 + t194) - C_CO * t199 - C_CO2 * t199 - C_H2 * t199 - C_CH4 * t199 - C_Tar * t199 - C_H2O * (-t197 + t205) - C_O2 * (-t208 + t198) - C_N2 * t199 + f_x(3,1);
t213 = 0.1e1 / x_norm_f_3 * t212;
t240 = 0.8017951980e4 * t25 * t73 * t49 * t65;
t241 = 0.1105875172e1 * t18;
t242 = 0.30000e5 * t103;
t245 = 0.30000e5 * t123;
t246 = -t245 - 0.7e-5;
t250 = 0.30000e5 * C_CO2 * t73 * t122;
t256 = 0.30000e5 * C_CH4 * t73 * t122;
t259 = 0.30000e5 * C_Tar * t73 * t122;
t262 = 0.30000e5 * C_H2O * t73 * t146;
t265 = 0.30000e5 * C_O2 * t73 * t122;
t268 = 0.30000e5 * C_N2 * t73 * t122;
t269 = -0.1831222341e-3 * t6 - t240 - T_s * (t241 - t242) - C_CO * t246 + t250 + 0.30000e5 * C_H2 * t73 * t122 + t256 + t259 + t262 + t265 + t268 + f_x(4,1);
t270 = 0.1e1 / x_norm_f_4 * t269;
t273 = 0.8017951980e4 * t76;
t288 = 0.30000e5 * t147;
t300 = t25 * t41 * t26 * t34;
t302 = 0.8017594994e1 * t18;
t303 = 0.120e3 * t90;
t307 = C_CO * t41 * t111;
t309 = 0.120e3 * t112;
t313 = C_H2 * t41 * t111;
t316 = C_CH4 * t41 * t111;
t319 = C_Tar * t41 * t111;
t322 = C_H2O * t41 * t111;
t328 = C_N2 * t41 * t111;
t330 = -0.1327636197e-2 * t6 - 0.3244122143e-5 * t300 - T_s * (t302 - t303) + 0.120e3 * t307 - C_CO2 * (-t309 - 0.7e-5) + 0.120e3 * t313 + 0.120e3 * t316 + 0.120e3 * t319 + 0.120e3 * t322 + 0.120e3 * C_O2 * t41 * t158 + 0.120e3 * t328 + f_x(5,1);
t331 = 0.1e1 / x_norm_f_5 * t330;
t359 = 0.1147345491e2 * t18;
t366 = -0.1899893179e-2 * t6 - t240 - T_s * (t359 - t242) + 0.30000e5 * C_CO * t73 * t122 + t250 - C_H2 * t246 + t256 + t259 + t262 + t265 + t268 + f_x(6,1);
t367 = 0.1e1 / x_norm_f_6 * t366;
t396 = 0.1e1 / x_norm_f_7 * (-0.1007172287e-2 * t6 - 0.6082313441e1 * t9 + 0.7e-5 * C_CH4 + f_x(7,1));
t410 = 0.1e1 / x_norm_f_8 * (-0.3153771810e-3 * t6 - 0.1904562796e1 * t9 + 0.7e-5 * C_Tar + f_x(8,1));
t421 = 0.2433091607e-6 * t46;
t422 = 0.7416605582e4 * t76;
t425 = 0.7602891803e1 * t18;
t426 = 0.9000e1 * t90;
t427 = 0.27750000e5 * t103;
t430 = 0.9000e1 * t112;
t431 = 0.27750000e5 * t123;
t432 = -t430 + t431;
t438 = 0.27750000e5 * t147;
t441 = 0.9000e1 * t159;
t445 = -0.1258965359e-2 * t6 - rho_char * (t421 - t422) - T_s * (t425 - t426 + t427) - C_CO * t432 - C_CO2 * t432 - C_H2 * t432 - C_CH4 * t432 - C_Tar * t432 - C_H2O * (-t430 + t438 - 0.7e-5) - C_O2 * (-t441 + t431) - C_N2 * t432 + f_x(9,1);
t446 = 0.1e1 / x_norm_f_9 * t445;
t483 = 0.12240e3 * t159;
t487 = 0.3309004586e-5 * t300 - 0.12240e3 * T_s * t41 * t89 - 0.12240e3 * t307 - 0.12240e3 * C_CO2 * t41 * t111 - 0.12240e3 * t313 - 0.12240e3 * t316 - 0.12240e3 * t319 - 0.12240e3 * t322 - C_O2 * (t483 - 0.7e-5) - 0.12240e3 * t328 + f_x(10,1);
t488 = 0.1e1 / x_norm_f_10 * t487;
t494 = 0.12240e3 * t112;
A_op(1,1) = -0.3000000000e0 * t3 + t12 * rho_coal;
A_op(1,2) = 0.0e0;
A_op(1,3) = -0.1811700000e4 * t18 + t12 * T_s;
A_op(1,4) = 0.0e0;
A_op(1,5) = 0.0e0;
A_op(1,6) = 0.0e0;
A_op(1,7) = 0.0e0;
A_op(1,8) = 0.0e0;
A_op(1,9) = 0.0e0;
A_op(1,10) = 0.0e0;
A_op(1,11) = 0.0e0;
A_op(2,1) = 0.2186484053e0 * t3 + t165 * rho_coal;
A_op(2,2) = t165 * rho_char - t47 - t77;
A_op(2,3) = t165 * T_s + t104 + t80 + t91;
A_op(2,4) = t165 * C_CO + t113 + t124;
A_op(2,5) = t165 * C_CO2 + t113 + t124;
A_op(2,6) = t165 * C_H2 + t113 + t124;
A_op(2,7) = t165 * C_CH4 + t113 + t124;
A_op(2,8) = t165 * C_Tar + t113 + t124;
A_op(2,9) = t165 * C_H2O + t113 + t148;
A_op(2,10) = t165 * C_O2 + t124 + t160;
A_op(2,11) = t165 * C_N2 + t113 + t124;
A_op(3,1) = 0.0e0;
A_op(3,2) = t213 * rho_char + t188 - t189;
A_op(3,3) = -0.1352813853e-3 - t193 + t194 + t213 * T_s;
A_op(3,4) = t213 * C_CO - t197 + t198;
A_op(3,5) = t213 * C_CO2 - t197 + t198;
A_op(3,6) = t213 * C_H2 - t197 + t198;
A_op(3,7) = t213 * C_CH4 - t197 + t198;
A_op(3,8) = t213 * C_Tar - t197 + t198;
A_op(3,9) = t213 * C_H2O - t197 + t205;
A_op(3,10) = t213 * C_O2 + t198 - t208;
A_op(3,11) = t213 * C_N2 - t197 + t198;
A_op(4,1) = 0.1831222341e-3 * t3 + t270 * rho_coal;
A_op(4,2) = t270 * rho_char + t273;
A_op(4,3) = t270 * T_s + t241 - t242;
A_op(4,4) = -t245 - 0.7e-5 + t270 * C_CO;
A_op(4,5) = t270 * C_CO2 - t245;
A_op(4,6) = t270 * C_H2 - t245;
A_op(4,7) = t270 * C_CH4 - t245;
A_op(4,8) = t270 * C_Tar - t245;
A_op(4,9) = t270 * C_H2O - t288;
A_op(4,10) = t270 * C_O2 - t245;
A_op(4,11) = t270 * C_N2 - t245;
A_op(5,1) = 0.1327636197e-2 * t3 + t331 * rho_coal;
A_op(5,2) = 0.3244122143e-5 * t46 + t331 * rho_char;
A_op(5,3) = t331 * T_s + t302 - t303;
A_op(5,4) = t331 * C_CO - t309;
A_op(5,5) = -t309 - 0.7e-5 + t331 * C_CO2;
A_op(5,6) = t331 * C_H2 - t309;
A_op(5,7) = t331 * C_CH4 - t309;
A_op(5,8) = t331 * C_Tar - t309;
A_op(5,9) = t331 * C_H2O - t309;
A_op(5,10) = t331 * C_O2 - 0.120e3 * t159;
A_op(5,11) = t331 * C_N2 - t309;
A_op(6,1) = 0.1899893179e-2 * t3 + t367 * rho_coal;
A_op(6,2) = t367 * rho_char + t273;
A_op(6,3) = t367 * T_s - t242 + t359;
A_op(6,4) = t367 * C_CO - t245;
A_op(6,5) = t367 * C_CO2 - t245;
A_op(6,6) = -t245 - 0.7e-5 + t367 * C_H2;
A_op(6,7) = t367 * C_CH4 - t245;
A_op(6,8) = t367 * C_Tar - t245;
A_op(6,9) = t367 * C_H2O - t288;
A_op(6,10) = t367 * C_O2 - t245;
A_op(6,11) = t367 * C_N2 - t245;
A_op(7,1) = 0.1007172287e-2 * t3 + t396 * rho_coal;
A_op(7,2) = 0.0e0;
A_op(7,3) = 0.6082313441e1 * t18 + t396 * T_s;
A_op(7,4) = 0.0e0;
A_op(7,5) = 0.0e0;
A_op(7,6) = 0.0e0;
A_op(7,7) = -0.7e-5 + t396 * C_CH4;
A_op(7,8) = 0.0e0;
A_op(7,9) = 0.0e0;
A_op(7,10) = 0.0e0;
A_op(7,11) = 0.0e0;
A_op(8,1) = 0.3153771810e-3 * t3 + t410 * rho_coal;
A_op(8,2) = 0.0e0;
A_op(8,3) = 0.1904562796e1 * t18 + t410 * T_s;
A_op(8,4) = 0.0e0;
A_op(8,5) = 0.0e0;
A_op(8,6) = 0.0e0;
A_op(8,7) = 0.0e0;
A_op(8,8) = -0.7e-5 + t410 * C_Tar;
A_op(8,9) = 0.0e0;
A_op(8,10) = 0.0e0;
A_op(8,11) = 0.0e0;
A_op(9,1) = 0.1258965359e-2 * t3 + t446 * rho_coal;
A_op(9,2) = t446 * rho_char + t421 - t422;
A_op(9,3) = t446 * T_s + t425 - t426 + t427;
A_op(9,4) = t446 * C_CO - t430 + t431;
A_op(9,5) = t446 * C_CO2 - t430 + t431;
A_op(9,6) = t446 * C_H2 - t430 + t431;
A_op(9,7) = t446 * C_CH4 - t430 + t431;
A_op(9,8) = t446 * C_Tar - t430 + t431;
A_op(9,9) = -t430 + t438 - 0.7e-5 + t446 * C_H2O;
A_op(9,10) = t446 * C_O2 + t431 - t441;
A_op(9,11) = t446 * C_N2 - t430 + t431;
A_op(10,1) = 0.0e0;
A_op(10,2) = -0.3309004586e-5 * t46 + t488 * rho_char;
A_op(10,3) = 0.12240e3 * t90 + t488 * T_s;
A_op(10,4) = t488 * C_CO + t494;
A_op(10,5) = t488 * C_CO2 + t494;
A_op(10,6) = t488 * C_H2 + t494;
A_op(10,7) = t488 * C_CH4 + t494;
A_op(10,8) = t488 * C_Tar + t494;
A_op(10,9) = t488 * C_H2O + t494;
A_op(10,10) = t483 - 0.7e-5 + t488 * C_O2;
A_op(10,11) = t488 * C_N2 + t494;
A_op(11,1) = 0.0e0;
A_op(11,2) = 0.0e0;
A_op(11,3) = 0.0e0;
A_op(11,4) = 0.0e0;
A_op(11,5) = 0.0e0;
A_op(11,6) = 0.0e0;
A_op(11,7) = 0.0e0;
A_op(11,8) = 0.0e0;
A_op(11,9) = 0.0e0;
A_op(11,10) = 0.0e0;
A_op(11,11) = -0.7e-5 + 0.1e1 / x_norm_f_11 * (0.7e-5 * C_N2 + f_x(11,1)) * C_N2;
 
%%
B_sys(1,1) = 0;
B_sys(1,2) = 0;
B_sys(2,1) = 0;
B_sys(2,2) = 0;
B_sys(3,1) = 0;
B_sys(3,2) = 0.1352813853e-3;
B_sys(4,1) = 0;
B_sys(4,2) = 0;
B_sys(5,1) = 0;
B_sys(5,2) = 0;
B_sys(6,1) = 0;
B_sys(6,2) = 0;
B_sys(7,1) = 0;
B_sys(7,2) = 0;
B_sys(8,1) = 0;
B_sys(8,2) = 0;
B_sys(9,1) = 0.7700000000e-2;
B_sys(9,2) = 0;
B_sys(10,1) = 0.1540000000e-2;
B_sys(10,2) = 0;
B_sys(11,1) = 0.7600000000e-3;
B_sys(11,2) = 0;
 
%%
t1 = C_CO + C_CO2 + C_H2 + C_CH4 + C_Tar + C_O2 + C_N2;
t2 = 0.1e1 / t1;
t4 = t1 ^ 2;
t5 = 0.1e1 / t4;
t7 = 0.2828e3 * C_CO * t5;
t9 = 0.2836e3 * C_H2 * t5;
t11 = 0.83616e3 * C_CH4 * t5;
t13 = -t7 - t9 - t11;
C_sys(1,1) = 0;
C_sys(1,2) = 0;
C_sys(1,3) = 0;
C_sys(1,4) = (0.2828e3 * t2 - t7 - t9 - t11);
C_sys(1,5) = t13;
C_sys(1,6) = (-t7 + 0.2836e3 * t2 - t9 - t11);
C_sys(1,7) = (-t7 - t9 + 0.83616e3 * t2 - t11);
C_sys(1,8) = t13;
C_sys(1,9) = 0;
C_sys(1,10) = t13;
C_sys(1,11) = t13;
  
 C_opt = C_sys+ ((HV-x'*C_sys')/(x'*x))*x';

%%%%%%%%%%%%
% y=C_opt*x;
a           =        A_op*Ts+eye(11,11);
b           =        B_sys(:,1)*Ts;
c           =        C_sys;
d           =        0;
%%%%%%%%%%%%%%%CALCULATING AUGMENTED MATRICES FOR MPC
[m1,n1] =  size(c);
[n1,n_in] =  size(b);
A_e =  eye(n1+m1,n1+m1);
A_e(1:n1,1:n1) = a;
A_e(n1+1:n1+m1,1:n1) =  c*a;
B_e =  zeros(n1+m1,n_in);
B_e(1:n1,:) = b;
B_e(n1+1:n1+m1,:) =  c*b;
C_e=zeros(m1,n1+m1);
C_e(:,n1+1:n1+m1) = eye(m1,m1);

Aa = A_e;
B = B_e;
C = C_e;
%
 dx_k_1 = A_op*x*Ts+eye(11,11)*x+B_sys(:,1)*u_k(1,1)*Ts+B_sys(:,2)*T*Ts;
 del_x  = dx_k_1-x;
%%%%%%%%%%%%%%%%%%%%%%%%%%%% Calculating Phi and F
 x_kn   = [del_x;y];


% % for 1e-3<delta_u<3e-3 and 0<u<5e-4 
% r_u=1*1.5;
% r_l=1*1.5;
% u_amp=5e-4;
% u_amp_l=1e-8;
r_u=.00000001*10.5;
r_l=.00000001*10.5;
u_amp=5e-4;
u_amp_l=0;
Aj=ones(Np,Np);
a1=tril(Aj);
Aj=ones(Np,Np);
a2=-tril(Aj);
a3=tril(Aj);
a4=-tril(Aj);
A_ineq=[a1;a2;a3;a4];
size(A_ineq);
b1=r_u*ones(Nc,1);
b2=r_l*ones(Nc,1);
b3=zeros(1,Nc);
b4=zeros(1,Nc);
b=zeros(4*Nc,1);
for i=1:Nc   
b3(i)=u_amp-u_k(i);
end
% u=u;
for i=1:Nc   
b4(i)=u_amp_l+u_k(i);
end
b=[b1;b2;b3';b4'];
size(b);

x_0 = Delta_U_k_1;
   [Delta_U,J] = MPC_UCG(x_0, A_ineq,b,x_kn, R_hat, R_s, Aa ,B, C, Np, Nc);

 u_k_1 = u_k+Delta_U;

%  toc
end

== matlab function UKF_MPCwithDISTandRefer/Unscented Kalman Filter UCG/Embedded MATLAB Function2 ==
  data: u input; y output
function y = fcn(u)
% This block supports the Embedded MATLAB subset.
% See the help menu for details. 

y = sqrt(diag(u));

== matlab function UKF_MPCwithDISTandRefer/Subsystem/MATLAB Function ==
  data: t input; y output; kurve parameter
function y = fcn(t,kurve)
%#codegen

     
persistent index  

if isempty(index) 
    index = 1;
end
a_4 = 0;
a_5 = 0;
a_6 = 0;
a_7 = 0;
t_0     = kurve(index,1);
t_f     = kurve(index,2);
x_t0    = kurve(index,3);
x_tf    = kurve(index,4);
dT      = t_f-t_0;
a_0     = x_t0;
if t >= t_0 && t < t_f        
a_4     = 35*(x_tf-x_t0)/dT^4;
a_5     = -84*(x_tf-x_t0)/dT^5;
a_6     = 70*(x_tf-x_t0)/dT^6;
a_7     = -20*(x_tf-x_t0)/dT^7;
end
%%
x_t     = a_0 + a_4*(t-t_0)^4 + a_5*(t-t_0)^5 + a_6*(t-t_0)^6 + a_7*(t-t_0)^7;
dx_dt   = 4*a_4*(t-t_0)^3 + 5*a_5*(t-t_0)^4 + 6*a_6*(t-t_0)^5 + 7*a_7*(t-t_0)^6;
dx2_dt  = 12*a_4*(t-t_0)^2 + 20*a_5*(t-t_0)^3 + 30*a_6*(t-t_0)^4 + 42*a_7*(t-t_0)^5;
dx3_dt  = 24*a_4*(t-t_0) + 60*a_5*(t-t_0)^2 + 120*a_6*(t-t_0)^3 + 210*a_7*(t-t_0)^4;
%%
if t >= t_0 + (t_f-t_0)
    x_t     = x_tf;
    dx_dt   = 0;
    dx2_dt  = 0;
    dx3_dt  = 0;
end

if index >= length(kurve)
    index = length(kurve)-1;
end
if t>kurve(index+1,1)
    index = index+1;
end
y = [x_t,dx_dt,dx2_dt,dx3_dt];

== matlab function UKF_MPCwithDISTandRefer/Unscented Kalman Filter UCG/Embedded MATLAB Function3 ==
  data: u input; y output
function y = fcn(u)
% This block supports the Embedded MATLAB subset.
% See the help menu for details. 

y = sqrt(diag(u));

== matlab function UKF_MPCwithDISTandRefer/Unscented Kalman Filter UCG/scaled output1 ==
  data: x input; HVukf output
function HVukf   = fcn(x)
Hco       = 282.8;          %KJ*mol-1, heat of combustion of CO
Hh2       = 283.6;          %KJ*mol-1, heat of combustion of H2
Hch4      = 836.16;         %KJ*mol-1, heat of combustion of CH4
CT=zeros(1,1);
yy=zeros(7,1);

%% Output matrix
C     = [0 0 0 1 0 0 0 0 0 0 0 
         0 0 0 0 1 0 0 0 0 0 0 
         0 0 0 0 0 1 0 0 0 0 0 
         0 0 0 0 0 0 1 0 0 0 0 
         0 0 0 0 0 0 0 1 0 0 0 
         0 0 0 0 0 0 0 0 0 1 0 
         0 0 0 0 0 0 0 0 0 0 1];
% y = C*x;
%% Adding noise to each output
% y =  [C_CO;C_CO2;C_H2;C_CH4;C_Tar;C_O2;C_N2] + v_noise;
y=C*x;
CT  = sum([y(1);y(2);y(3);y(4);y(5);y(6);y(7)]);
HVukf=zeros(1,1);
HVukf  = Hco*y(1)/CT+Hh2*y(3)/CT+Hch4*y(4)/CT;

== matlab function UKF_MPCwithDISTandRefer/UCG Plant/MATLAB Function ==
  data: w input; y output
function y = fcn(w)
%#codegen
y = w*ones(11,1);

== matlab function UKF_MPCwithDISTandRefer/MPC UCG/MATLAB Function1 ==
  data: t input; u input; y output
function y = fcn(t,u)
%#codegen
if t<20000
    y=2e-4;
else
y = 1*u;
end

== matlab function UKF_MPCwithDISTandRefer/UCG Plant/scaled output ==
  data: y_meas input; y_scaled output; y_max parameter; y_min parameter
function y_scaled   = fcn(y_meas,y_max, y_min)
%#codegen
% rho_coal = x(1);
% rho_char = x(2);
% T_s      = x(3);
% C_CO     = x(4);
% C_CO2    = x(5);
% C_H2     = x(6);
% C_CH4    = x(7);
% C_Tar    = x(8);
% C_H2O    = x(9);
% C_O2     = x(10);
% C_N2     = x(11);

% y =  [C_CO;C_CO2;C_H2;C_CH4;C_Tar;C_O2;C_N2] + v_noise;
%% %%%%%%%%%%%%%%%%%%%%%
y_scaled = zeros(7,1);
for i=1:length(y_scaled)
y_scaled(i) = (y_meas(i)-y_min(i))./(y_max(i)-y_min(i));
% y_scaled_full=[rho_coal;rho_char;T_s;C_H2O;C_CO;C_CO2;C_H2;C_CH4;C_Tar;C_O2;C_N2]'
end
% y_scaled=y_scaled_full(5:11,:);

== matlab function UKF_MPCwithDISTandRefer/Subsystem/Error_mpc ==
  data: error_mpc output; Ref input; HV input
function error_mpc = fcn(Ref,HV)
%#codegen
% l=t;
error_mpc=Ref-HV;

== matlab function UKF_MPCwithDISTandRefer/UCG Plant/State output splitter ==
  data: rn1 input; rn2 input; u input; HVm output; ym output
% function [z,HVm,ym,ym_wo_noise] = fcn(rn1,rn2,u)
function [HVm,ym] = fcn(rn1,rn2,u)
%#codegen
% ym_wo_noise=zeros(7,1);
% z = [u(1);u(2); u(3); u(9)];
ym = [u(4) ;u(5); u(6) ;u(7); u(8); u(10); u(11)];
% ym_wo_noise=ym;
ym1 = [ym(1);ym(3);ym(4)];
ym2 = [ym(2);ym(5);ym(6);ym(7)];

ym1 =ym1*rn1+ym1;
ym2 =ym2*rn2+ym2;

%ym = rn*ym+ym;
ym =[ym1(1);ym2(1);ym1(2);ym1(3);ym2(2);ym2(3);ym2(4)];

Hco       = 282.8;          %KJ*mol-1, heat of combustion of CO
Hh2       = 283.6;          %KJ*mol-1, heat of combustion of H2
Hch4      = 836.16;         %KJ*mol-1, heat of combustion of CH4
CT  = sum([ym1;ym2]);

HVm  = Hco*ym1(1)/CT+Hh2*ym1(2)/CT+Hch4*ym1(3)/CT;
